simulink model "trackMove"  (Simulink 8.6)
settings: Solver=VariableStepAuto  StartTime=t_start  StopTime=t_end  MaxStep=0.0000001  RelTol=1e-3  AbsTol=0.0000001
values from neighbouring files (symbols this model uses):
  delay1 = 0.001+0.001*k    [singleAntennaProgram.m]    (also in trackMoveEdit.m = 0.02+0.02*k)
  delay2 = 0.0014+0.001*k    [singleAntennaProgram.m]    (also in trackMoveEdit.m = 0.06+0.02*k)
libraries: dsparch4 x4, simulink x3, commchan3 x2, commsynccomp2 x1
settings Model: Creator=my88899  LastModifiedBy=my88899
settings SolverCC: InitialStep=0.0000001
settings DataIOCC: SaveFormat=Dataset  SignalLoggingSaveFormat=Dataset
settings OptimizationCC: ExpressionDepthLimit=128
settings DebuggingCC: UnderspecifiedInitializationDetection=Simplified  MergeDetectMultiDrivingBlocksExec=error  SolverPrmCheckMsg=none  FcnCallInpInsideContextMsg=EnableAllAsError  StateNameClashWarn=none
settings HardwareCC: ProdBitPerPointer=64  ProdLargestAtomicFloat=Float  ProdIntDivRoundTo=Zero  ProdEndianess=LittleEndian  ProdWordSize=64  ProdHWDeviceType=Intel->x86-64 (Windows64)
settings GRTTargetCC: GeneratePreprocessorConditionals=Use local settings  CombineOutputUpdateFcns=on  GRTInterface=off
settings ConfigComp: CovModelRefEnable=off

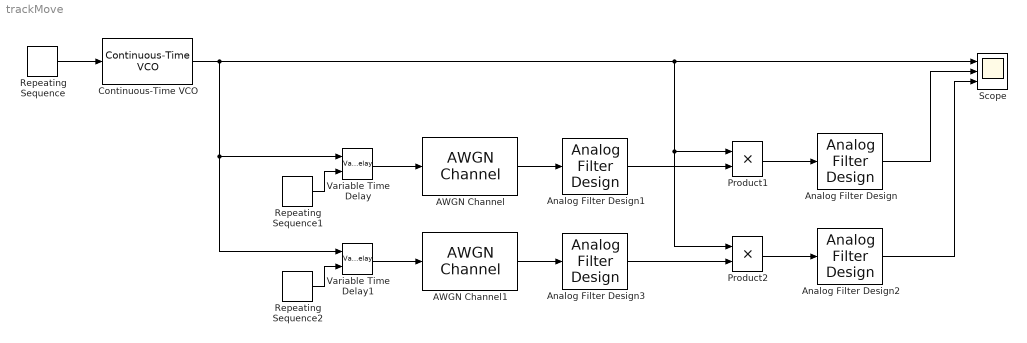
== system trackMove ==
  AWGN Channel : commchan3/AWGN Channel  InputProcessing=Columns as channels (frame based)  seed=67  noiseMode=Variance from mask  EbNodB=10  EsNodB=10  SNRdB=10  bitsPerSym=1  Ps=1  Tsym=1000000  variance=1
  AWGN Channel1 : commchan3/AWGN Channel  InputProcessing=Columns as channels (frame based)  seed=67  noiseMode=Variance from mask  EbNodB=10  EsNodB=10  SNRdB=10  bitsPerSym=1  Ps=1  Tsym=1000000  variance=1
  Analog Filter Design : dsparch4/Analog Filter Design  method=Butterworth  filttype=Lowpass  N=12  Wlo=2*pi*30000  Whi=80  Rp=2  Rs=40
  Analog Filter Design1 : dsparch4/Analog Filter Design  method=Butterworth  filttype=Highpass  N=12  Wlo=2*pi*10000  Whi=80  Rp=2  Rs=40
  Analog Filter Design2 : dsparch4/Analog Filter Design  method=Butterworth  filttype=Lowpass  N=12  Wlo=2*pi*30000  Whi=80  Rp=2  Rs=40
  Analog Filter Design3 : dsparch4/Analog Filter Design  method=Butterworth  filttype=Highpass  N=12  Wlo=2*pi*10000  Whi=80  Rp=2  Rs=40
  Continuous-Time VCO : commsynccomp2/Continuous-Time VCO  Ac=5  Fc=100000  Kc=10000  Ph=0
  Product1 : Product
  Product2 : Product
  Repeating Sequence : simulink/Sources/Repeating Sequence  rep_seq_t=[0 1]  rep_seq_y=[0 10]
  Repeating Sequence1 : simulink/Sources/Repeating Sequence  rep_seq_t=[0 1]  rep_seq_y=[delay1 delay2]
  Repeating Sequence2 : simulink/Sources/Repeating Sequence  rep_seq_t=[0 1]  rep_seq_y=[delay1 delay2]
  Scope : Scope  NumInputPorts=3
  Variable Time Delay : VariableTransportDelay  MaximumDelay=0.5  MaximumPoints=5000448
  Variable Time Delay1 : VariableTransportDelay  MaximumDelay=0.5  MaximumPoints=5000448
  wires:
  Repeating Sequence/1 -> Continuous-Time VCO/1
  Variable Time Delay/1 -> AWGN Channel/1
  Analog Filter Design1/1 -> Product1/2
  AWGN Channel/1 -> Analog Filter Design1/1
  Repeating Sequence1/1 -> Variable Time Delay/2
  Product1/1 -> Analog Filter Design/1
  Analog Filter Design/1 -> Scope/2
  Variable Time Delay1/1 -> AWGN Channel1/1
  Analog Filter Design3/1 -> Product2/2
  AWGN Channel1/1 -> Analog Filter Design3/1
  Repeating Sequence2/1 -> Variable Time Delay1/2
  Product2/1 -> Analog Filter Design2/1
  Analog Filter Design2/1 -> Scope/3
  Continuous-Time VCO/1 -> Variable Time Delay1/1, Variable Time Delay/1, Product2/1, Product1/1, Scope/1
